simulink library "lib_rfsoc_fec"  (R2020b)
settings: Solver=VariableStepAuto  StartTime=0.0  StopTime=10.0  RelTol=1e-3
undefined symbols (not defined in the file): d, fs, generator_polynomial
libraries: commseqgen3 x84, hdlsllib x83, $bdroot x33, simulink x22, dspsigops x13
(part 2 of 4)

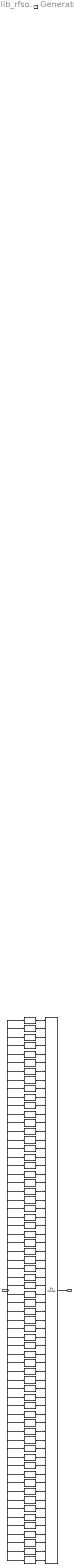
== system lib_rfsoc_fec/Random Number Generator/Random Number Generator ==
  reset : Inport
  enable : EnablePort
  bit0 : commseqgen3/PN Sequence Generator  poly='z^13 + z^12 + z^11 + z^8 + 1'  ini_sta=[ 1 1 1 0 0 1 1 0 0 1 1 0 0]  outBitMaskSource=Dialog parameter  shift=0  outVarSiz=off  maxOutSizeMode=Dialog parameter  maxOutSize=[10 1]  Ts=-1  sampPerFrame=1  reset=on  bitPackedOutputs=off  outDataType=boolean  numPackedBits=8  bitPackDataSigned=off  bitPackedOutDType=double
  bit1 : commseqgen3/PN Sequence Generator  poly='z^13 + z^12 + z^11 + z^8 + 1'  ini_sta=[ 1 0 0 0 0 1 1 0 0 0 1 0 1]  outBitMaskSource=Dialog parameter  shift=0  outVarSiz=off  maxOutSizeMode=Dialog parameter  maxOutSize=[10 1]  Ts=-1  sampPerFrame=1  reset=on  bitPackedOutputs=off  outDataType=boolean  numPackedBits=8  bitPackDataSigned=off  bitPackedOutDType=double
  bit10 : commseqgen3/PN Sequence Generator  poly='z^13 + z^12 + z^11 + z^8 + 1'  ini_sta=[ 1 0 1 0 0 0 1 1 0 1 1 0 0]  outBitMaskSource=Dialog parameter  shift=0  outVarSiz=off  maxOutSizeMode=Dialog parameter  maxOutSize=[10 1]  Ts=-1  sampPerFrame=1  reset=on  bitPackedOutputs=off  outDataType=boolean  numPackedBits=8  bitPackDataSigned=off  bitPackedOutDType=double
  bit11 : commseqgen3/PN Sequence Generator  poly='z^13 + z^12 + z^11 + z^8 + 1'  ini_sta=[ 0 1 0 1 0 1 1 1 1 1 0 1 0]  outBitMaskSource=Dialog parameter  shift=0  outVarSiz=off  maxOutSizeMode=Dialog parameter  maxOutSize=[10 1]  Ts=-1  sampPerFrame=1  reset=on  bitPackedOutputs=off  outDataType=boolean  numPackedBits=8  bitPackDataSigned=off  bitPackedOutDType=double
  bit12 : commseqgen3/PN Sequence Generator  poly='z^13 + z^12 + z^11 + z^8 + 1'  ini_sta=[ 0 0 1 1 0 1 1 1 0 1 1 1 0]  outBitMaskSource=Dialog parameter  shift=0  outVarSiz=off  maxOutSizeMode=Dialog parameter  maxOutSize=[10 1]  Ts=-1  sampPerFrame=1  reset=on  bitPackedOutputs=off  outDataType=boolean  numPackedBits=8  bitPackDataSigned=off  bitPackedOutDType=double
  bit13 : commseqgen3/PN Sequence Generator  poly='z^13 + z^12 + z^11 + z^8 + 1'  ini_sta=[ 1 1 0 0 1 0 0 1 0 1 0 0 0]  outBitMaskSource=Dialog parameter  shift=0  outVarSiz=off  maxOutSizeMode=Dialog parameter  maxOutSize=[10 1]  Ts=-1  sampPerFrame=1  reset=on  bitPackedOutputs=off  outDataType=boolean  numPackedBits=8  bitPackDataSigned=off  bitPackedOutDType=double
  bit14 : commseqgen3/PN Sequence Generator  poly='z^13 + z^12 + z^11 + z^8 + 1'  ini_sta=[ 1 0 1 1 1 0 0 1 0 0 0 1 1]  outBitMaskSource=Dialog parameter  shift=0  outVarSiz=off  maxOutSizeMode=Dialog parameter  maxOutSize=[10 1]  Ts=-1  sampPerFrame=1  reset=on  bitPackedOutputs=off  outDataType=boolean  numPackedBits=8  bitPackDataSigned=off  bitPackedOutDType=double
  bit15 : commseqgen3/PN Sequence Generator  poly='z^13 + z^12 + z^11 + z^8 + 1'  ini_sta=[ 0 1 0 0 0 1 1 1 0 1 1 0 0]  outBitMaskSource=Dialog parameter  shift=0  outVarSiz=off  maxOutSizeMode=Dialog parameter  maxOutSize=[10 1]  Ts=-1  sampPerFrame=1  reset=on  bitPackedOutputs=off  outDataType=boolean  numPackedBits=8  bitPackDataSigned=off  bitPackedOutDType=double
  bit16 : commseqgen3/PN Sequence Generator  poly='z^13 + z^12 + z^11 + z^8 + 1'  ini_sta=[ 1 0 0 1 0 1 0 1 0 0 0 1 1]  outBitMaskSource=Dialog parameter  shift=0  outVarSiz=off  maxOutSizeMode=Dialog parameter  maxOutSize=[10 1]  Ts=-1  sampPerFrame=1  reset=on  bitPackedOutputs=off  outDataType=boolean  numPackedBits=8  bitPackDataSigned=off  bitPackedOutDType=double
  bit17 : commseqgen3/PN Sequence Generator  poly='z^13 + z^12 + z^11 + z^8 + 1'  ini_sta=[ 0 1 1 0 1 0 1 1 1 1 0 0 1]  outBitMaskSource=Dialog parameter  shift=0  outVarSiz=off  maxOutSizeMode=Dialog parameter  maxOutSize=[10 1]  Ts=-1  sampPerFrame=1  reset=on  bitPackedOutputs=off  outDataType=boolean  numPackedBits=8  bitPackDataSigned=off  bitPackedOutDType=double
  bit18 : commseqgen3/PN Sequence Generator  poly='z^13 + z^12 + z^11 + z^8 + 1'  ini_sta=[ 0 0 0 1 0 1 1 1 1 0 0 1 1]  outBitMaskSource=Dialog parameter  shift=0  outVarSiz=off  maxOutSizeMode=Dialog parameter  maxOutSize=[10 1]  Ts=-1  sampPerFrame=1  reset=on  bitPackedOutputs=off  outDataType=boolean  numPackedBits=8  bitPackDataSigned=off  bitPackedOutDType=double
  bit19 : commseqgen3/PN Sequence Generator  poly='z^13 + z^12 + z^11 + z^8 + 1'  ini_sta=[ 0 0 0 0 0 1 1 0 0 0 1 0 1]  outBitMaskSource=Dialog parameter  shift=0  outVarSiz=off  maxOutSizeMode=Dialog parameter  maxOutSize=[10 1]  Ts=-1  sampPerFrame=1  reset=on  bitPackedOutputs=off  outDataType=boolean  numPackedBits=8  bitPackDataSigned=off  bitPackedOutDType=double
  bit2 : commseqgen3/PN Sequence Generator  poly='z^13 + z^12 + z^11 + z^8 + 1'  ini_sta=[ 0 0 0 1 1 1 1 0 1 1 0 0 1]  outBitMaskSource=Dialog parameter  shift=0  outVarSiz=off  maxOutSizeMode=Dialog parameter  maxOutSize=[10 1]  Ts=-1  sampPerFrame=1  reset=on  bitPackedOutputs=off  outDataType=boolean  numPackedBits=8  bitPackDataSigned=off  bitPackedOutDType=double
  bit20 : commseqgen3/PN Sequence Generator  poly='z^13 + z^12 + z^11 + z^8 + 1'  ini_sta=[ 0 1 1 1 1 1 0 1 1 0 1 1 1]  outBitMaskSource=Dialog parameter  shift=0  outVarSiz=off  maxOutSizeMode=Dialog parameter  maxOutSize=[10 1]  Ts=-1  sampPerFrame=1  reset=on  bitPackedOutputs=off  outDataType=boolean  numPackedBits=8  bitPackDataSigned=off  bitPackedOutDType=double
  bit21 : commseqgen3/PN Sequence Generator  poly='z^13 + z^12 + z^11 + z^8 + 1'  ini_sta=[ 0 1 0 0 0 1 1 1 0 1 0 0 0]  outBitMaskSource=Dialog parameter  shift=0  outVarSiz=off  maxOutSizeMode=Dialog parameter  maxOutSize=[10 1]  Ts=-1  sampPerFrame=1  reset=on  bitPackedOutputs=off  outDataType=boolean  numPackedBits=8  bitPackDataSigned=off  bitPackedOutDType=double
  bit22 : commseqgen3/PN Sequence Generator  poly='z^13 + z^12 + z^11 + z^8 + 1'  ini_sta=[ 0 1 0 1 0 1 1 0 1 1 1 1 1]  outBitMaskSource=Dialog parameter  shift=0  outVarSiz=off  maxOutSizeMode=Dialog parameter  maxOutSize=[10 1]  Ts=-1  sampPerFrame=1  reset=on  bitPackedOutputs=off  outDataType=boolean  numPackedBits=8  bitPackDataSigned=off  bitPackedOutDType=double
  bit23 : commseqgen3/PN Sequence Generator  poly='z^13 + z^12 + z^11 + z^8 + 1'  ini_sta=[ 0 1 0 0 1 0 0 1 1 0 0 1 0]  outBitMaskSource=Dialog parameter  shift=0  outVarSiz=off  maxOutSizeMode=Dialog parameter  maxOutSize=[10 1]  Ts=-1  sampPerFrame=1  reset=on  bitPackedOutputs=off  outDataType=boolean  numPackedBits=8  bitPackDataSigned=off  bitPackedOutDType=double
  bit24 : commseqgen3/PN Sequence Generator  poly='z^13 + z^12 + z^11 + z^8 + 1'  ini_sta=[ 0 0 1 0 1 0 1 1 1 1 0 0 0]  outBitMaskSource=Dialog parameter  shift=0  outVarSiz=off  maxOutSizeMode=Dialog parameter  maxOutSize=[10 1]  Ts=-1  sampPerFrame=1  reset=on  bitPackedOutputs=off  outDataType=boolean  numPackedBits=8  bitPackDataSigned=off  bitPackedOutDType=double
  bit25 : commseqgen3/PN Sequence Generator  poly='z^13 + z^12 + z^11 + z^8 + 1'  ini_sta=[ 0 1 1 0 0 1 1 0 0 0 1 1 1]  outBitMaskSource=Dialog parameter  shift=0  outVarSiz=off  maxOutSizeMode=Dialog parameter  maxOutSize=[10 1]  Ts=-1  sampPerFrame=1  reset=on  bitPackedOutputs=off  outDataType=boolean  numPackedBits=8  bitPackDataSigned=off  bitPackedOutDType=double
  bit26 : commseqgen3/PN Sequence Generator  poly='z^13 + z^12 + z^11 + z^8 + 1'  ini_sta=[ 1 0 1 1 0 0 1 0 1 0 0 1 1]  outBitMaskSource=Dialog parameter  shift=0  outVarSiz=off  maxOutSizeMode=Dialog parameter  maxOutSize=[10 1]  Ts=-1  sampPerFrame=1  reset=on  bitPackedOutputs=off  outDataType=boolean  numPackedBits=8  bitPackDataSigned=off  bitPackedOutDType=double
  bit27 : commseqgen3/PN Sequence Generator  poly='z^13 + z^12 + z^11 + z^8 + 1'  ini_sta=[ 0 0 1 1 0 1 0 0 0 0 1 0 1]  outBitMaskSource=Dialog parameter  shift=0  outVarSiz=off  maxOutSizeMode=Dialog parameter  maxOutSize=[10 1]  Ts=-1  sampPerFrame=1  reset=on  bitPackedOutputs=off  outDataType=boolean  numPackedBits=8  bitPackDataSigned=off  bitPackedOutDType=double
  bit28 : commseqgen3/PN Sequence Generator  poly='z^13 + z^12 + z^11 + z^8 + 1'  ini_sta=[ 1 0 1 0 1 0 1 0 1 0 0 1 0]  outBitMaskSource=Dialog parameter  shift=0  outVarSiz=off  maxOutSizeMode=Dialog parameter  maxOutSize=[10 1]  Ts=-1  sampPerFrame=1  reset=on  bitPackedOutputs=off  outDataType=boolean  numPackedBits=8  bitPackDataSigned=off  bitPackedOutDType=double
  bit29 : commseqgen3/PN Sequence Generator  poly='z^13 + z^12 + z^11 + z^8 + 1'  ini_sta=[ 0 1 1 1 0 0 0 1 0 1 1 1 0]  outBitMaskSource=Dialog parameter  shift=0  outVarSiz=off  maxOutSizeMode=Dialog parameter  maxOutSize=[10 1]  Ts=-1  sampPerFrame=1  reset=on  bitPackedOutputs=off  outDataType=boolean  numPackedBits=8  bitPackDataSigned=off  bitPackedOutDType=double
  bit3 : commseqgen3/PN Sequence Generator  poly='z^13 + z^12 + z^11 + z^8 + 1'  ini_sta=[ 0 0 1 0 1 1 0 1 1 0 0 0 1]  outBitMaskSource=Dialog parameter  shift=0  outVarSiz=off  maxOutSizeMode=Dialog parameter  maxOutSize=[10 1]  Ts=-1  sampPerFrame=1  reset=on  bitPackedOutputs=off  outDataType=boolean  numPackedBits=8  bitPackDataSigned=off  bitPackedOutDType=double
  bit30 : commseqgen3/PN Sequence Generator  poly='z^13 + z^12 + z^11 + z^8 + 1'  ini_sta=[ 0 1 1 0 1 1 1 0 1 1 1 1 0]  outBitMaskSource=Dialog parameter  shift=0  outVarSiz=off  maxOutSizeMode=Dialog parameter  maxOutSize=[10 1]  Ts=-1  sampPerFrame=1  reset=on  bitPackedOutputs=off  outDataType=boolean  numPackedBits=8  bitPackDataSigned=off  bitPackedOutDType=double
  bit31 : commseqgen3/PN Sequence Generator  poly='z^13 + z^12 + z^11 + z^8 + 1'  ini_sta=[ 0 0 1 0 1 1 0 0 1 1 1 0 0]  outBitMaskSource=Dialog parameter  shift=0  outVarSiz=off  maxOutSizeMode=Dialog parameter  maxOutSize=[10 1]  Ts=-1  sampPerFrame=1  reset=on  bitPackedOutputs=off  outDataType=boolean  numPackedBits=8  bitPackDataSigned=off  bitPackedOutDType=double
  bit32 : commseqgen3/PN Sequence Generator  poly='z^13 + z^12 + z^11 + z^8 + 1'  ini_sta=[ 0 0 1 1 0 0 0 1 0 1 1 1 1]  outBitMaskSource=Dialog parameter  shift=0  outVarSiz=off  maxOutSizeMode=Dialog parameter  maxOutSize=[10 1]  Ts=-1  sampPerFrame=1  reset=on  bitPackedOutputs=off  outDataType=boolean  numPackedBits=8  bitPackDataSigned=off  bitPackedOutDType=double
  bit33 : commseqgen3/PN Sequence Generator  poly='z^13 + z^12 + z^11 + z^8 + 1'  ini_sta=[ 1 0 0 1 1 1 0 1 1 1 0 1 0]  outBitMaskSource=Dialog parameter  shift=0  outVarSiz=off  maxOutSizeMode=Dialog parameter  maxOutSize=[10 1]  Ts=-1  sampPerFrame=1  reset=on  bitPackedOutputs=off  outDataType=boolean  numPackedBits=8  bitPackDataSigned=off  bitPackedOutDType=double
  bit34 : commseqgen3/PN Sequence Generator  poly='z^13 + z^12 + z^11 + z^8 + 1'  ini_sta=[ 0 1 0 0 0 1 0 0 1 1 1 0 0]  outBitMaskSource=Dialog parameter  shift=0  outVarSiz=off  maxOutSizeMode=Dialog parameter  maxOutSize=[10 1]  Ts=-1  sampPerFrame=1  reset=on  bitPackedOutputs=off  outDataType=boolean  numPackedBits=8  bitPackDataSigned=off  bitPackedOutDType=double
  bit35 : commseqgen3/PN Sequence Generator  poly='z^13 + z^12 + z^11 + z^8 + 1'  ini_sta=[ 1 0 0 0 1 1 1 1 0 1 0 0 1]  outBitMaskSource=Dialog parameter  shift=0  outVarSiz=off  maxOutSizeMode=Dialog parameter  maxOutSize=[10 1]  Ts=-1  sampPerFrame=1  reset=on  bitPackedOutputs=off  outDataType=boolean  numPackedBits=8  bitPackDataSigned=off  bitPackedOutDType=double
  bit36 : commseqgen3/PN Sequence Generator  poly='z^13 + z^12 + z^11 + z^8 + 1'  ini_sta=[ 1 1 1 1 0 0 0 1 1 1 0 1 1]  outBitMaskSource=Dialog parameter  shift=0  outVarSiz=off  maxOutSizeMode=Dialog parameter  maxOutSize=[10 1]  Ts=-1  sampPerFrame=1  reset=on  bitPackedOutputs=off  outDataType=boolean  numPackedBits=8  bitPackDataSigned=off  bitPackedOutDType=double
  bit37 : commseqgen3/PN Sequence Generator  poly='z^13 + z^12 + z^11 + z^8 + 1'  ini_sta=[ 1 0 1 1 0 1 1 0 1 1 1 0 1]  outBitMaskSource=Dialog parameter  shift=0  outVarSiz=off  maxOutSizeMode=Dialog parameter  maxOutSize=[10 1]  Ts=-1  sampPerFrame=1  reset=on  bitPackedOutputs=off  outDataType=boolean  numPackedBits=8  bitPackDataSigned=off  bitPackedOutDType=double
  bit38 : commseqgen3/PN Sequence Generator  poly='z^13 + z^12 + z^11 + z^8 + 1'  ini_sta=[ 1 0 1 0 1 1 0 1 1 1 1 0 0]  outBitMaskSource=Dialog parameter  shift=0  outVarSiz=off  maxOutSizeMode=Dialog parameter  maxOutSize=[10 1]  Ts=-1  sampPerFrame=1  reset=on  bitPackedOutputs=off  outDataType=boolean  numPackedBits=8  bitPackDataSigned=off  bitPackedOutDType=double
  bit39 : commseqgen3/PN Sequence Generator  poly='z^13 + z^12 + z^11 + z^8 + 1'  ini_sta=[ 1 1 1 1 0 1 0 1 1 0 0 1 1]  outBitMaskSource=Dialog parameter  shift=0  outVarSiz=off  maxOutSizeMode=Dialog parameter  maxOutSize=[10 1]  Ts=-1  sampPerFrame=1  reset=on  bitPackedOutputs=off  outDataType=boolean  numPackedBits=8  bitPackDataSigned=off  bitPackedOutDType=double
  bit4 : commseqgen3/PN Sequence Generator  poly='z^13 + z^12 + z^11 + z^8 + 1'  ini_sta=[ 1 0 1 1 0 1 0 0 1 1 0 0 0]  outBitMaskSource=Dialog parameter  shift=0  outVarSiz=off  maxOutSizeMode=Dialog parameter  maxOutSize=[10 1]  Ts=-1  sampPerFrame=1  reset=on  bitPackedOutputs=off  outDataType=boolean  numPackedBits=8  bitPackDataSigned=off  bitPackedOutDType=double
  bit40 : commseqgen3/PN Sequence Generator  poly='z^13 + z^12 + z^11 + z^8 + 1'  ini_sta=[ 1 1 0 0 0 1 1 0 0 1 1 1 1]  outBitMaskSource=Dialog parameter  shift=0  outVarSiz=off  maxOutSizeMode=Dialog parameter  maxOutSize=[10 1]  Ts=-1  sampPerFrame=1  reset=on  bitPackedOutputs=off  outDataType=boolean  numPackedBits=8  bitPackDataSigned=off  bitPackedOutDType=double
  bit41 : commseqgen3/PN Sequence Generator  poly='z^13 + z^12 + z^11 + z^8 + 1'  ini_sta=[ 1 0 0 1 1 0 1 1 1 0 0 1 0]  outBitMaskSource=Dialog parameter  shift=0  outVarSiz=off  maxOutSizeMode=Dialog parameter  maxOutSize=[10 1]  Ts=-1  sampPerFrame=1  reset=on  bitPackedOutputs=off  outDataType=boolean  numPackedBits=8  bitPackDataSigned=off  bitPackedOutDType=double
  bit42 : commseqgen3/PN Sequence Generator  poly='z^13 + z^12 + z^11 + z^8 + 1'  ini_sta=[ 1 1 1 1 0 0 1 0 1 0 1 1 0]  outBitMaskSource=Dialog parameter  shift=0  outVarSiz=off  maxOutSizeMode=Dialog parameter  maxOutSize=[10 1]  Ts=-1  sampPerFrame=1  reset=on  bitPackedOutputs=off  outDataType=boolean  numPackedBits=8  bitPackDataSigned=off  bitPackedOutDType=double
  bit43 : commseqgen3/PN Sequence Generator  poly='z^13 + z^12 + z^11 + z^8 + 1'  ini_sta=[ 0 0 0 0 1 1 1 1 0 1 0 0 1]  outBitMaskSource=Dialog parameter  shift=0  outVarSiz=off  maxOutSizeMode=Dialog parameter  maxOutSize=[10 1]  Ts=-1  sampPerFrame=1  reset=on  bitPackedOutputs=off  outDataType=boolean  numPackedBits=8  bitPackDataSigned=off  bitPackedOutDType=double
  bit44 : commseqgen3/PN Sequence Generator  poly='z^13 + z^12 + z^11 + z^8 + 1'  ini_sta=[ 0 1 0 0 0 1 0 0 1 1 0 1 0]  outBitMaskSource=Dialog parameter  shift=0  outVarSiz=off  maxOutSizeMode=Dialog parameter  maxOutSize=[10 1]  Ts=-1  sampPerFrame=1  reset=on  bitPackedOutputs=off  outDataType=boolean  numPackedBits=8  bitPackDataSigned=off  bitPackedOutDType=double
  bit45 : commseqgen3/PN Sequence Generator  poly='z^13 + z^12 + z^11 + z^8 + 1'  ini_sta=[ 1 1 1 1 1 1 0 0 1 0 0 1 0]  outBitMaskSource=Dialog parameter  shift=0  outVarSiz=off  maxOutSizeMode=Dialog parameter  maxOutSize=[10 1]  Ts=-1  sampPerFrame=1  reset=on  bitPackedOutputs=off  outDataType=boolean  numPackedBits=8  bitPackDataSigned=off  bitPackedOutDType=double
  bit46 : commseqgen3/PN Sequence Generator  poly='z^13 + z^12 + z^11 + z^8 + 1'  ini_sta=[ 1 1 0 0 0 1 0 1 1 0 1 1 0]  outBitMaskSource=Dialog parameter  shift=0  outVarSiz=off  maxOutSizeMode=Dialog parameter  maxOutSize=[10 1]  Ts=-1  sampPerFrame=1  reset=on  bitPackedOutputs=off  outDataType=boolean  numPackedBits=8  bitPackDataSigned=off  bitPackedOutDType=double
  bit47 : commseqgen3/PN Sequence Generator  poly='z^13 + z^12 + z^11 + z^8 + 1'  ini_sta=[ 0 1 1 1 1 0 0 1 1 0 1 1 0]  outBitMaskSource=Dialog parameter  shift=0  outVarSiz=off  maxOutSizeMode=Dialog parameter  maxOutSize=[10 1]  Ts=-1  sampPerFrame=1  reset=on  bitPackedOutputs=off  outDataType=boolean  numPackedBits=8  bitPackDataSigned=off  bitPackedOutDType=double
  bit48 : commseqgen3/PN Sequence Generator  poly='z^13 + z^12 + z^11 + z^8 + 1'  ini_sta=[ 1 0 1 0 1 1 1 0 0 1 0 1 0]  outBitMaskSource=Dialog parameter  shift=0  outVarSiz=off  maxOutSizeMode=Dialog parameter  maxOutSize=[10 1]  Ts=-1  sampPerFrame=1  reset=on  bitPackedOutputs=off  outDataType=boolean  numPackedBits=8  bitPackDataSigned=off  bitPackedOutDType=double
  bit49 : commseqgen3/PN Sequence Generator  poly='z^13 + z^12 + z^11 + z^8 + 1'  ini_sta=[ 0 1 1 0 1 0 1 0 1 1 0 0 0]  outBitMaskSource=Dialog parameter  shift=0  outVarSiz=off  maxOutSizeMode=Dialog parameter  maxOutSize=[10 1]  Ts=-1  sampPerFrame=1  reset=on  bitPackedOutputs=off  outDataType=boolean  numPackedBits=8  bitPackDataSigned=off  bitPackedOutDType=double
  bit5 : commseqgen3/PN Sequence Generator  poly='z^13 + z^12 + z^11 + z^8 + 1'  ini_sta=[ 1 1 0 1 0 1 0 0 1 1 0 1 0]  outBitMaskSource=Dialog parameter  shift=0  outVarSiz=off  maxOutSizeMode=Dialog parameter  maxOutSize=[10 1]  Ts=-1  sampPerFrame=1  reset=on  bitPackedOutputs=off  outDataType=boolean  numPackedBits=8  bitPackDataSigned=off  bitPackedOutDType=double
  bit50 : commseqgen3/PN Sequence Generator  poly='z^13 + z^12 + z^11 + z^8 + 1'  ini_sta=[ 0 1 1 0 0 0 0 1 0 1 0 1 0]  outBitMaskSource=Dialog parameter  shift=0  outVarSiz=off  maxOutSizeMode=Dialog parameter  maxOutSize=[10 1]  Ts=-1  sampPerFrame=1  reset=on  bitPackedOutputs=off  outDataType=boolean  numPackedBits=8  bitPackDataSigned=off  bitPackedOutDType=double
  bit51 : commseqgen3/PN Sequence Generator  poly='z^13 + z^12 + z^11 + z^8 + 1'  ini_sta=[ 0 0 1 1 0 1 1 0 1 0 0 1 1]  outBitMaskSource=Dialog parameter  shift=0  outVarSiz=off  maxOutSizeMode=Dialog parameter  maxOutSize=[10 1]  Ts=-1  sampPerFrame=1  reset=on  bitPackedOutputs=off  outDataType=boolean  numPackedBits=8  bitPackDataSigned=off  bitPackedOutDType=double
  bit52 : commseqgen3/PN Sequence Generator  poly='z^13 + z^12 + z^11 + z^8 + 1'  ini_sta=[ 0 1 1 0 0 0 1 0 0 0 0 0 1]  outBitMaskSource=Dialog parameter  shift=0  outVarSiz=off  maxOutSizeMode=Dialog parameter  maxOutSize=[10 1]  Ts=-1  sampPerFrame=1  reset=on  bitPackedOutputs=off  outDataType=boolean  numPackedBits=8  bitPackDataSigned=off  bitPackedOutDType=double
  bit53 : commseqgen3/PN Sequence Generator  poly='z^13 + z^12 + z^11 + z^8 + 1'  ini_sta=[ 0 0 0 0 0 1 1 1 1 0 1 0 0]  outBitMaskSource=Dialog parameter  shift=0  outVarSiz=off  maxOutSizeMode=Dialog parameter  maxOutSize=[10 1]  Ts=-1  sampPerFrame=1  reset=on  bitPackedOutputs=off  outDataType=boolean  numPackedBits=8  bitPackDataSigned=off  bitPackedOutDType=double
  bit54 : commseqgen3/PN Sequence Generator  poly='z^13 + z^12 + z^11 + z^8 + 1'  ini_sta=[ 0 1 1 1 1 0 0 0 1 1 1 0 1]  outBitMaskSource=Dialog parameter  shift=0  outVarSiz=off  maxOutSizeMode=Dialog parameter  maxOutSize=[10 1]  Ts=-1  sampPerFrame=1  reset=on  bitPackedOutputs=off  outDataType=boolean  numPackedBits=8  bitPackDataSigned=off  bitPackedOutDType=double
  bit55 : commseqgen3/PN Sequence Generator  poly='z^13 + z^12 + z^11 + z^8 + 1'  ini_sta=[ 0 1 0 1 0 1 0 1 0 1 0 1 1]  outBitMaskSource=Dialog parameter  shift=0  outVarSiz=off  maxOutSizeMode=Dialog parameter  maxOutSize=[10 1]  Ts=-1  sampPerFrame=1  reset=on  bitPackedOutputs=off  outDataType=boolean  numPackedBits=8  bitPackDataSigned=off  bitPackedOutDType=double
  bit56 : commseqgen3/PN Sequence Generator  poly='z^13 + z^12 + z^11 + z^8 + 1'  ini_sta=[ 1 1 1 1 1 0 0 1 1 1 0 1 0]  outBitMaskSource=Dialog parameter  shift=0  outVarSiz=off  maxOutSizeMode=Dialog parameter  maxOutSize=[10 1]  Ts=-1  sampPerFrame=1  reset=on  bitPackedOutputs=off  outDataType=boolean  numPackedBits=8  bitPackDataSigned=off  bitPackedOutDType=double
  bit57 : commseqgen3/PN Sequence Generator  poly='z^13 + z^12 + z^11 + z^8 + 1'  ini_sta=[ 1 0 0 0 1 1 1 0 0 0 1 1 0]  outBitMaskSource=Dialog parameter  shift=0  outVarSiz=off  maxOutSizeMode=Dialog parameter  maxOutSize=[10 1]  Ts=-1  sampPerFrame=1  reset=on  bitPackedOutputs=off  outDataType=boolean  numPackedBits=8  bitPackDataSigned=off  bitPackedOutDType=double
  bit58 : commseqgen3/PN Sequence Generator  poly='z^13 + z^12 + z^11 + z^8 + 1'  ini_sta=[ 1 1 0 1 1 0 0 0 1 0 1 0 1]  outBitMaskSource=Dialog parameter  shift=0  outVarSiz=off  maxOutSizeMode=Dialog parameter  maxOutSize=[10 1]  Ts=-1  sampPerFrame=1  reset=on  bitPackedOutputs=off  outDataType=boolean  numPackedBits=8  bitPackDataSigned=off  bitPackedOutDType=double
  bit59 : commseqgen3/PN Sequence Generator  poly='z^13 + z^12 + z^11 + z^8 + 1'  ini_sta=[ 0 1 1 0 1 0 0 0 0 1 1 1 1]  outBitMaskSource=Dialog parameter  shift=0  outVarSiz=off  maxOutSizeMode=Dialog parameter  maxOutSize=[10 1]  Ts=-1  sampPerFrame=1  reset=on  bitPackedOutputs=off  outDataType=boolean  numPackedBits=8  bitPackDataSigned=off  bitPackedOutDType=double
  bit6 : commseqgen3/PN Sequence Generator  poly='z^13 + z^12 + z^11 + z^8 + 1'  ini_sta=[ 0 0 0 0 1 0 0 0 1 1 1 1 0]  outBitMaskSource=Dialog parameter  shift=0  outVarSiz=off  maxOutSizeMode=Dialog parameter  maxOutSize=[10 1]  Ts=-1  sampPerFrame=1  reset=on  bitPackedOutputs=off  outDataType=boolean  numPackedBits=8  bitPackDataSigned=off  bitPackedOutDType=double
  bit60 : commseqgen3/PN Sequence Generator  poly='z^13 + z^12 + z^11 + z^8 + 1'  ini_sta=[ 0 1 1 1 0 1 1 0 0 1 0 0 1]  outBitMaskSource=Dialog parameter  shift=0  outVarSiz=off  maxOutSizeMode=Dialog parameter  maxOutSize=[10 1]  Ts=-1  sampPerFrame=1  reset=on  bitPackedOutputs=off  outDataType=boolean  numPackedBits=8  bitPackDataSigned=off  bitPackedOutDType=double
  bit61 : commseqgen3/PN Sequence Generator  poly='z^13 + z^12 + z^11 + z^8 + 1'  ini_sta=[ 1 1 0 1 0 0 1 1 1 0 0 0 1]  outBitMaskSource=Dialog parameter  shift=0  outVarSiz=off  maxOutSizeMode=Dialog parameter  maxOutSize=[10 1]  Ts=-1  sampPerFrame=1  reset=on  bitPackedOutputs=off  outDataType=boolean  numPackedBits=8  bitPackDataSigned=off  bitPackedOutDType=double
  bit62 : commseqgen3/PN Sequence Generator  poly='z^13 + z^12 + z^11 + z^8 + 1'  ini_sta=[ 1 1 1 1 1 1 0 1 1 0 1 1 1]  outBitMaskSource=Dialog parameter  shift=0  outVarSiz=off  maxOutSizeMode=Dialog parameter  maxOutSize=[10 1]  Ts=-1  sampPerFrame=1  reset=on  bitPackedOutputs=off  outDataType=boolean  numPackedBits=8  bitPackDataSigned=off  bitPackedOutDType=double
  bit63 : commseqgen3/PN Sequence Generator  poly='z^13 + z^12 + z^11 + z^8 + 1'  ini_sta=[ 1 0 0 0 0 1 1 0 0 0 1 0 0]  outBitMaskSource=Dialog parameter  shift=0  outVarSiz=off  maxOutSizeMode=Dialog parameter  maxOutSize=[10 1]  Ts=-1  sampPerFrame=1  reset=on  bitPackedOutputs=off  outDataType=boolean  numPackedBits=8  bitPackDataSigned=off  bitPackedOutDType=double
  bit7 : commseqgen3/PN Sequence Generator  poly='z^13 + z^12 + z^11 + z^8 + 1'  ini_sta=[ 1 1 0 0 0 0 1 0 0 0 0 0 0]  outBitMaskSource=Dialog parameter  shift=0  outVarSiz=off  maxOutSizeMode=Dialog parameter  maxOutSize=[10 1]  Ts=-1  sampPerFrame=1  reset=on  bitPackedOutputs=off  outDataType=boolean  numPackedBits=8  bitPackDataSigned=off  bitPackedOutDType=double
  bit8 : commseqgen3/PN Sequence Generator  poly='z^13 + z^12 + z^11 + z^8 + 1'  ini_sta=[ 1 1 1 1 0 1 0 1 0 0 0 0 0]  outBitMaskSource=Dialog parameter  shift=0  outVarSiz=off  maxOutSizeMode=Dialog parameter  maxOutSize=[10 1]  Ts=-1  sampPerFrame=1  reset=on  bitPackedOutputs=off  outDataType=boolean  numPackedBits=8  bitPackDataSigned=off  bitPackedOutDType=double
  bit9 : commseqgen3/PN Sequence Generator  poly='z^13 + z^12 + z^11 + z^8 + 1'  ini_sta=[ 0 1 0 1 0 1 1 1 1 1 0 0 1]  outBitMaskSource=Dialog parameter  shift=0  outVarSiz=off  maxOutSizeMode=Dialog parameter  maxOutSize=[10 1]  Ts=-1  sampPerFrame=1  reset=on  bitPackedOutputs=off  outDataType=boolean  numPackedBits=8  bitPackDataSigned=off  bitPackedOutDType=double
  concat : hdlsllib/Logic and Bit Operations/Bit Concat  numInputs=64
  data : Outport
  wires:
  concat/1 -> data/1
  bit63/1 -> concat/64
  bit62/1 -> concat/63
  bit61/1 -> concat/62
  bit60/1 -> concat/61
  bit59/1 -> concat/60
  bit58/1 -> concat/59
  bit57/1 -> concat/58
  bit56/1 -> concat/57
  bit55/1 -> concat/56
  bit54/1 -> concat/55
  bit53/1 -> concat/54
  bit52/1 -> concat/53
  bit51/1 -> concat/52
  bit50/1 -> concat/51
  bit49/1 -> concat/50
  bit48/1 -> concat/49
  bit47/1 -> concat/48
  bit46/1 -> concat/47
  bit45/1 -> concat/46
  bit44/1 -> concat/45
  bit43/1 -> concat/44
  bit42/1 -> concat/43
  bit41/1 -> concat/42
  bit40/1 -> concat/41
  bit39/1 -> concat/40
  bit38/1 -> concat/39
  bit37/1 -> concat/38
  bit36/1 -> concat/37
  bit35/1 -> concat/36
  bit34/1 -> concat/35
  bit33/1 -> concat/34
  bit32/1 -> concat/33
  bit31/1 -> concat/32
  bit30/1 -> concat/31
  bit29/1 -> concat/30
  bit28/1 -> concat/29
  bit27/1 -> concat/28
  bit26/1 -> concat/27
  bit25/1 -> concat/26
  bit24/1 -> concat/25
  bit23/1 -> concat/24
  bit22/1 -> concat/23
  bit21/1 -> concat/22
  bit20/1 -> concat/21
  bit19/1 -> concat/20
  bit18/1 -> concat/19
  bit17/1 -> concat/18
  bit16/1 -> concat/17
  bit15/1 -> concat/16
  bit14/1 -> concat/15
  bit13/1 -> concat/14
  bit12/1 -> concat/13
  bit11/1 -> concat/12
  bit10/1 -> concat/11
  bit9/1 -> concat/10
  bit8/1 -> concat/9
  bit7/1 -> concat/8
  bit6/1 -> concat/7
  bit5/1 -> concat/6
  bit4/1 -> concat/5
  bit3/1 -> concat/4
  bit2/1 -> concat/3
  bit1/1 -> concat/2
  bit0/1 -> concat/1
  reset/1 -> bit63/1, bit62/1, bit61/1, bit60/1, bit59/1, bit58/1, bit57/1, bit56/1, bit55/1, bit54/1, bit53/1, bit52/1, bit51/1, bit50/1, bit49/1, bit48/1, bit47/1, bit46/1, bit45/1, bit44/1, bit43/1, bit42/1, bit41/1, bit40/1, bit39/1, bit38/1, bit37/1, bit36/1, bit35/1, bit34/1, bit33/1, bit32/1, bit31/1, bit30/1, bit29/1, bit28/1, bit27/1, bit26/1, bit25/1, bit24/1, bit23/1, bit22/1, bit21/1, bit20/1, bit19/1, bit18/1, bit17/1, bit16/1, bit15/1, bit14/1, bit13/1, bit12/1, bit11/1, bit10/1, bit9/1, bit8/1, bit7/1, bit6/1, bit5/1, bit4/1, bit3/1, bit2/1, bit1/1, bit0/1

== system lib_rfsoc_fec/Random Number Generator/byte_count ==
  reset : Inport
  en : Inport  Port=2
  Cast To Boolean : DataTypeConversion  OutDataTypeStr=boolean
  Delay3 : Delay  DelayLength=1
  Delay5 : Delay  DelayLength=1
  HDL Counter : hdlsllib/Sources/HDL Counter  CountType=Count limited  CountInit=0  CountStep=1  CountMax=1  CountFromType=Initial value  CountFrom=0  CountResetPort=on  CountLoadPort=off  CountEnbPort=on  CountDirPort=off  CountDataType=Unsigned  CountWordLen=1  CountFracLen=0  CountSampTime=1
  HDL Counter1 : hdlsllib/Sources/HDL Counter  CountType=Count limited  CountInit=0  CountStep=1  CountMax=3  CountFromType=Initial value  CountFrom=0  CountResetPort=on  CountLoadPort=off  CountEnbPort=on  CountDirPort=off  CountDataType=Unsigned  CountWordLen=2  CountFracLen=0  CountSampTime=1
  OR : Logic  Operator=OR  IconShape=distinctive  AllPortsSameDT=off  OutDataTypeStr=boolean
  falling_edge : Subsystem
  count : Outport
  valid : Outport  Port=2
  wires:
  Cast To Boolean/1 -> HDL Counter1/2, valid/1
  falling_edge/1(pulse) -> OR/2
  Delay3/1 -> OR/1
  HDL Counter1/1 -> count/1
  reset/1 -> Delay3/1
  Delay5/1 -> HDL Counter/2, falling_edge/1(in)
  HDL Counter/1 -> Cast To Boolean/1
  OR/1 -> HDL Counter/1, HDL Counter1/1
  en/1 -> Delay5/1

== system lib_rfsoc_fec/Random Number Generator/concat ==
  en : Inport
  d_in : Inport  Port=2
  diff : Inport  Port=3
  Bit Concat : hdlsllib/Logic and Bit Operations/Bit Concat  numInputs=2
  Bitwise Operator : simulink/Logic and Bit Operations/Bitwise Operator  logicop=AND  UseBitMask=off  NumInputPorts=2  BitMask=bin2dec('11011001')  BitMaskRealWorld=Stored Integer
  Constant : Constant  Value=0  OutDataTypeStr=fixdt(0,128,0)  SampleTime=-1
  Delay : Delay  DelayLength=1
  Delay1 : Delay  DelayLength=1
  Delay4 : Delay  DelayLength=1
  Multiport Switch : MultiPortSwitch  DataPortOrder=Zero-based contiguous  Inputs=2  zeroidx=on
  mask_generator : Subsystem
  d_out : Outport
  wires:
  Delay/1 -> Multiport Switch/1
  Constant/1 -> Multiport Switch/2
  Bitwise Operator/1 -> Multiport Switch/3
  en/1 -> mask_generator/2(sel), Delay/1
  Multiport Switch/1 -> d_out/1
  mask_generator/1(mask) -> Bitwise Operator/2
  Delay1/1 -> Bitwise Operator/1
  diff/1 -> mask_generator/1(diff)
  Bit Concat/1 -> Delay1/1
  d_in/1 -> Delay4/1, Bit Concat/1
  Delay4/1 -> Bit Concat/2

== system lib_rfsoc_fec/Random Number Generator/hold for multiple of 4 ==
  In1 : Inport
  Compare To Constant : simulink/Logic and Bit Operations/Compare To Constant  relop===  const=7  OutDataTypeStr=boolean
  HDL Counter : hdlsllib/Sources/HDL Counter  CountType=Count limited  CountInit=0  CountStep=1  CountMax=7  CountFromType=Initial value  CountFrom=0  CountResetPort=off  CountLoadPort=off  CountEnbPort=on  CountDirPort=off  CountDataType=Unsigned  CountWordLen=3  CountFracLen=0  CountSampTime=1
  OR : Logic  Operator=OR  IconShape=distinctive  AllPortsSameDT=off  OutDataTypeStr=boolean
  Sample and Hold1 : dspsigops/Sample and Hold  trig=Rising edge  initCond=0  latchinput=off
  " " : Outport
  wires:
  Compare To Constant/1 -> OR/1
  HDL Counter/1 -> Compare To Constant/1
  OR/1 -> Sample and Hold1/Trigger
  Sample and Hold1/1 -> " "/1, HDL Counter/1
  In1/1 -> Sample and Hold1/1, OR/2

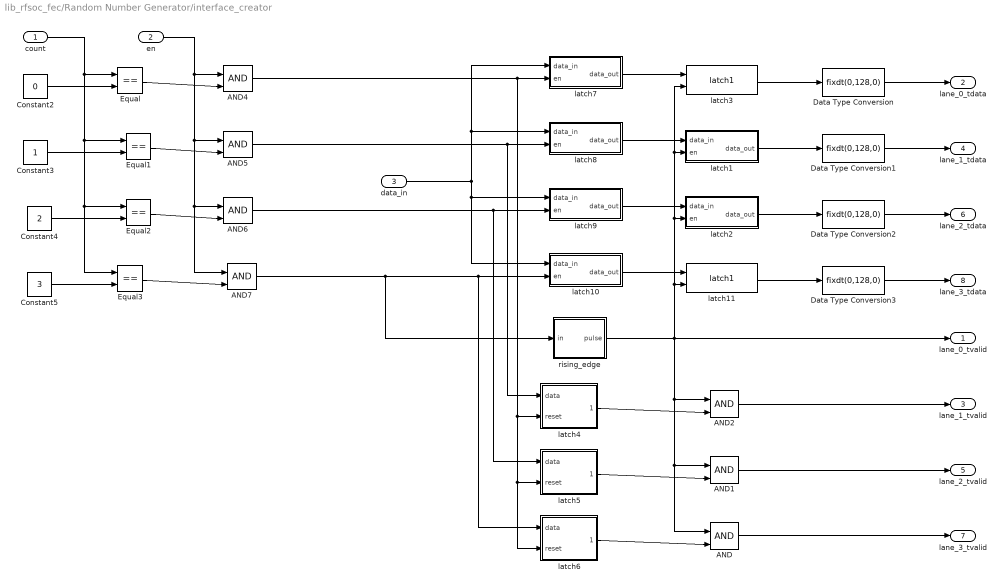
== system lib_rfsoc_fec/Random Number Generator/interface_creator ==
  count : Inport
  en : Inport  Port=2
  data_in : Inport  Port=3
  AND{,1..2,4..7} (7 alike) : Logic  IconShape=distinctive  AllPortsSameDT=off  OutDataTypeStr=boolean
  Constant2 : Constant  Value=0  OutDataTypeStr=fixdt(0,2,0)  SampleTime=-1
  Constant3 : Constant  OutDataTypeStr=fixdt(0,2,0)  SampleTime=-1
  Constant4 : Constant  Value=2  OutDataTypeStr=fixdt(0,2,0)  SampleTime=-1
  Constant5 : Constant  Value=3  OutDataTypeStr=fixdt(0,2,0)  SampleTime=-1
  Data Type Conversion{,1..3} (4 alike) : DataTypeConversion  OutDataTypeStr=fixdt(0,128,0)
  Equal{,1..3} (4 alike) : RelationalOperator  Operator===  OutDataTypeStr=boolean  RndMeth=Simplest
  latch1 : Subsystem
  latch10 : Subsystem
  latch11 : $bdroot/Random Number Generator/interface_creator/latch1  SystemSampleTime=-1  VariantActivationTime=update diagram  Latency=0  AutoFrameSizeCalculation=off
  latch2 : Subsystem
  latch3 : $bdroot/Random Number Generator/interface_creator/latch1  SystemSampleTime=-1  VariantActivationTime=update diagram  Latency=0  AutoFrameSizeCalculation=off
  latch4 : Subsystem
  latch5 : Subsystem
  latch6 : Subsystem
  latch7 : Subsystem
  latch8 : Subsystem
  latch9 : Subsystem
  rising_edge : Subsystem
  lane_0_tvalid : Outport
  lane_0_tdata : Outport  Port=2
  lane_1_tvalid : Outport  Port=3
  lane_1_tdata : Outport  Port=4
  lane_2_tvalid : Outport  Port=5
  lane_2_tdata : Outport  Port=6
  lane_3_tvalid : Outport  Port=7
  lane_3_tdata : Outport  Port=8
  wires:
  AND/1 -> lane_3_tvalid/1
  latch2/1(data_out) -> Data Type Conversion2/1
  latch6/1(data_out) -> AND/2
  AND7/1 -> latch6/1(data), latch10/2(en), rising_edge/1(in)
  latch4/1(data_out) -> AND2/2
  Constant3/1 -> Equal1/2
  latch10/1(data_out) -> latch11/1
  latch1/1(data_out) -> Data Type Conversion1/1
  Equal/1 -> AND4/2
  Equal1/1 -> AND5/2
  latch5/1(data_out) -> AND1/2
  AND1/1 -> lane_2_tvalid/1
  Equal2/1 -> AND6/2
  rising_edge/1(pulse) -> AND2/1, AND1/1, AND/1, latch11/2, latch2/2(en), latch3/2, latch1/2(en), lane_0_tvalid/1
  Constant2/1 -> Equal/2
  latch11/1 -> Data Type Conversion3/1
  latch7/1(data_out) -> latch3/1
  AND4/1 -> latch7/2(en), latch4/2(reset), latch5/2(reset), latch6/2(reset)
  latch9/1(data_out) -> latch2/1(data_in)
  en/1 -> AND4/1, AND7/1, AND6/1, AND5/1
  Constant5/1 -> Equal3/2
  Constant4/1 -> Equal2/2
  AND5/1 -> latch4/1(data), latch8/2(en)
  AND6/1 -> latch5/1(data), latch9/2(en)
  AND2/1 -> lane_1_tvalid/1
  latch8/1(data_out) -> latch1/1(data_in)
  data_in/1 -> latch8/1(data_in), latch7/1(data_in), latch9/1(data_in), latch10/1(data_in)
  latch3/1 -> Data Type Conversion/1
  Equal3/1 -> AND7/2
  count/1 -> Equal/1, Equal1/1, Equal2/1, Equal3/1
  Data Type Conversion/1 -> lane_0_tdata/1
  Data Type Conversion1/1 -> lane_1_tdata/1
  Data Type Conversion2/1 -> lane_2_tdata/1
  Data Type Conversion3/1 -> lane_3_tdata/1

== system lib_rfsoc_fec/Random Number Generator/rising_edge ==
  in : Inport
  Data Type Conversion1 : DataTypeConversion  OutDataTypeStr=boolean  SaturateOnIntegerOverflow=on  RndMeth=Zero
  Delay15 : Delay  DelayLength=1  InitialCondition=1  InputProcessing=Columns as channels (frame based)
  Logical Operator2 : Logic  Operator=NOT  Inputs=1
  Logical Operator3 : Logic
  pulse : Outport
  wires:
  Logical Operator2/1 -> Logical Operator3/2
  in/1 -> Data Type Conversion1/1
  Data Type Conversion1/1 -> Logical Operator3/1, Delay15/1
  Logical Operator3/1 -> pulse/1
  Delay15/1 -> Logical Operator2/1

== system lib_rfsoc_fec/Random Number Generator/tvalid hold ==
  trigger : Inport
  comparator : Inport  Port=2
  Cast To Boolean : DataTypeConversion  OutDataTypeStr=boolean
  Delay2 : Delay  DelayLength=1
  Equal : RelationalOperator  OutDataTypeStr=boolean  RndMeth=Simplest
  HDL Counter : hdlsllib/Sources/HDL Counter  CountType=Free running  CountInit=0  CountStep=128  CountMax=25  CountFromType=Initial value  CountFrom=0  CountResetPort=on  CountLoadPort=off  CountEnbPort=on  CountDirPort=off  CountDataType=Unsigned  CountWordLen=32  CountFracLen=0  CountSampTime=1
  HDL Counter1 : hdlsllib/Sources/HDL Counter  CountType=Count limited  CountInit=0  CountStep=1  CountMax=1  CountFromType=Initial value  CountFrom=0  CountResetPort=on  CountLoadPort=off  CountEnbPort=on  CountDirPort=off  CountDataType=Unsigned  CountWordLen=1  CountFracLen=0  CountSampTime=1
  Multiport Switch : MultiPortSwitch  DataPortOrder=Zero-based contiguous  Inputs=2  zeroidx=on
  OR : Logic  Operator=OR  IconShape=distinctive  AllPortsSameDT=off  OutDataTypeStr=boolean
  Subtract : Sum  Inputs=+-
  enable : Outport
  diff : Outport  Port=2
  wires:
  Cast To Boolean/1 -> HDL Counter/2
  HDL Counter1/1 -> Cast To Boolean/1
  Subtract/1 -> diff/1
  HDL Counter/1 -> Equal/1, Subtract/1
  Equal/1 -> HDL Counter/1, HDL Counter1/1, OR/1
  trigger/1 -> Multiport Switch/3, OR/2
  comparator/1 -> Equal/2, Subtract/2
  Multiport Switch/1 -> Delay2/1, HDL Counter1/2, enable/1
  Delay2/1 -> Multiport Switch/2
  OR/1 -> Multiport Switch/1

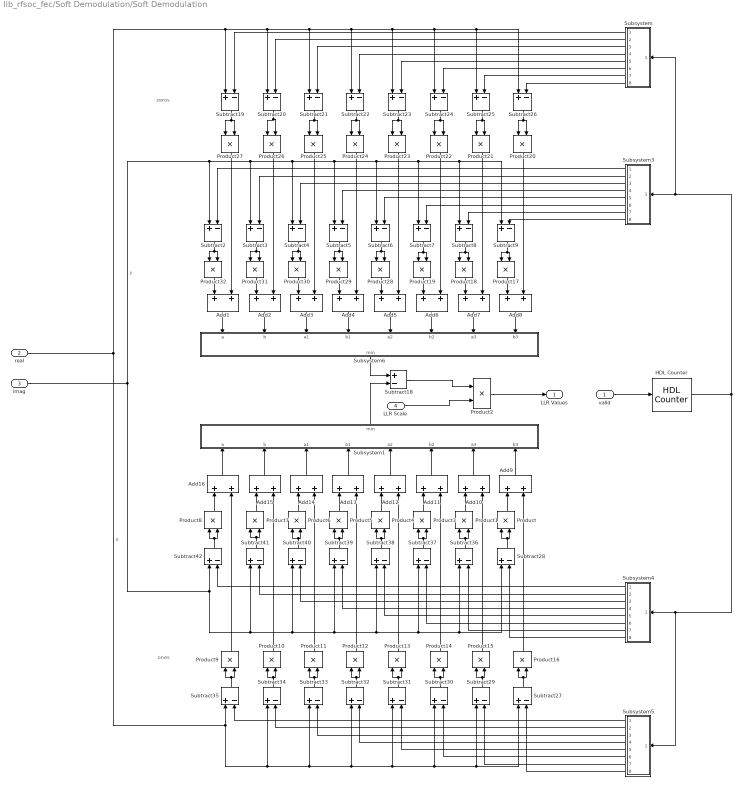
== system lib_rfsoc_fec/Soft Demodulation/Soft Demodulation ==
  note: ones
  note: zeros
  valid : Inport
  real : Inport  Port=2
  imag : Inport  Port=3
  LLR Scale : Inport  Port=4
  Add{1..16} (16 alike) : Sum  OutDataTypeStr=fixdt(1,35,22)  SaturateOnIntegerOverflow=on
  HDL Counter : hdlsllib/Sources/HDL Counter  CountType=Count limited  CountInit=0  CountStep=1  CountMax=3  CountFromType=Initial value  CountFrom=0  CountResetPort=off  CountLoadPort=off  CountEnbPort=on  CountDirPort=off  CountDataType=Unsigned  CountWordLen=2  CountFracLen=0  CountSampTime=1/(fs*2)
  Product{,1,3..16} (16 alike) : Product  SaturateOnIntegerOverflow=on
  Product{17..32} (16 alike) : Product
  Product2 : Product  OutDataTypeStr=fixdt(1,24,12)  RndMeth=Round  SaturateOnIntegerOverflow=on
  Subsystem : Subsystem
  Subsystem1 : Subsystem
  Subsystem3 : Subsystem
  Subsystem4 : Subsystem
  Subsystem5 : Subsystem
  Subsystem6 : Subsystem
  Subtract18 : Sum  Inputs=+-  OutDataTypeStr=fixdt(1,35,22)  SaturateOnIntegerOverflow=on
  Subtract{2..9,19..42} (32 alike) : Sum  Inputs=+-  OutDataTypeStr=fixdt(1,17,11)  SaturateOnIntegerOverflow=on
  LLR Values : Outport
  wires:
  HDL Counter/1 -> Subsystem3/1(enb), Subsystem/1(enb), Subsystem4/1(enb), Subsystem5/1(enb)
  valid/1 -> HDL Counter/1
  Subsystem/8(Out8) -> Subtract26/2
  Subsystem/7(Out7) -> Subtract25/2
  Subsystem/6(Out6) -> Subtract24/2
  Subsystem/5(Out5) -> Subtract23/2
  Subsystem/4(Out4) -> Subtract22/2
  Subsystem/3(Out3) -> Subtract21/2
  Subsystem/2(Out2) -> Subtract20/2
  Subsystem/1(Out1) -> Subtract19/2
  Subtract7/1 -> Product19/2, Product19/1
  Subtract22/1 -> Product24/2, Product24/1
  Subtract20/1 -> Product26/1, Product26/2
  Subtract8/1 -> Product18/2, Product18/1
  Subtract9/1 -> Product17/1, Product17/2
  Subtract27/1 -> Product16/2, Product16/1
  Subtract29/1 -> Product15/2, Product15/1
  Subtract30/1 -> Product14/2, Product14/1
  Subtract31/1 -> Product13/2, Product13/1
  Subtract32/1 -> Product12/2, Product12/1
  Subtract33/1 -> Product11/2, Product11/1
  Subtract37/1 -> Product3/2, Product3/1
  Product2/1 -> LLR Values/1
  Subsystem5/5(Out5) -> Subtract31/2
  Subtract28/1 -> Product/1, Product/2
  Add5/1 -> Subsystem6/5(a2)
  Subsystem3/8(Out8) -> Subtract9/2
  Add4/1 -> Subsystem6/4(b1)
  Product11/1 -> Add14/2
  Product29/1 -> Add4/1
  Subsystem4/8(Out8) -> Subtract28/2
  Subsystem4/2(Out2) -> Subtract41/2
  Subsystem5/8(Out8) -> Subtract27/2
  Subsystem5/7(Out7) -> Subtract29/2
  Subtract40/1 -> Product6/1, Product6/2
  Subtract34/1 -> Product10/1, Product10/2
  Product32/1 -> Add1/1
  Subsystem5/1(Out1) -> Subtract35/2
  Subtract39/1 -> Product5/1, Product5/2
  Subsystem3/7(Out7) -> Subtract8/2
  Product16/1 -> Add9/2
  Subsystem4/1(Out1) -> Subtract42/2
  Subsystem5/6(Out6) -> Subtract30/2
  Product24/1 -> Add4/2
  Subtract3/1 -> Product31/2, Product31/1
  Product13/1 -> Add12/2
  Subsystem5/3(Out3) -> Subtract33/2
  Subsystem5/2(Out2) -> Subtract34/2
  Subsystem4/3(Out3) -> Subtract40/2
  Product17/1 -> Add8/1
  Subsystem4/4(Out4) -> Subtract39/2
  Product9/1 -> Add16/2
  Add15/1 -> Subsystem1/2(b)
  Subsystem4/7(Out7) -> Subtract36/2
  Subtract26/1 -> Product20/2, Product20/1
  Subsystem3/3(Out3) -> Subtract4/2
  Product28/1 -> Add5/1
  Product12/1 -> Add13/2
  Product8/1 -> Add16/1
  Product7/1 -> Add15/1
  Subsystem4/5(Out5) -> Subtract38/2
  Subsystem3/4(Out4) -> Subtract5/2
  Product21/1 -> Add7/2
  Subtract25/1 -> Product21/2, Product21/1
  Add6/1 -> Subsystem6/6(b2)
  Add13/1 -> Subsystem1/4(b1)
  Add2/1 -> Subsystem6/2(b)
  Product15/1 -> Add10/2
  Product14/1 -> Add11/2
  Add8/1 -> Subsystem6/8(b3)
  Product27/1 -> Add1/2
  Subsystem3/1(Out1) -> Subtract2/2
  Subtract42/1 -> Product8/1, Product8/2
  Subtract36/1 -> Product1/1, Product1/2
  Subtract23/1 -> Product23/1, Product23/2
  Add10/1 -> Subsystem1/7(a3)
  imag/1 -> Subtract42/1, Subtract39/1, Subtract28/1, Subtract36/1, Subtract37/1, Subtract38/1, Subtract40/1, Subtract41/1, Subtract9/1, Subtract8/1, Subtract7/1, Subtract6/1, Subtract5/1, Subtract4/1, Subtract3/1, Subtract2/1  "y"
  Add16/1 -> Subsystem1/1(a)
  Subtract2/1 -> Product32/2, Product32/1
  Subtract6/1 -> Product28/2, Product28/1
  Subtract5/1 -> Product29/1, Product29/2
  Product18/1 -> Add7/1
  Add9/1 -> Subsystem1/8(b3)
  Product30/1 -> Add3/1
  Subsystem3/5(Out5) -> Subtract6/2
  Product31/1 -> Add2/1
  Subtract19/1 -> Product27/2, Product27/1
  Product26/1 -> Add2/2
  Add11/1 -> Subsystem1/6(b2)
  Subsystem3/2(Out2) -> Subtract3/2
  Product22/1 -> Add6/2
  Subsystem1/1(min) -> Subtract18/2
  Product5/1 -> Add13/1
  Subtract18/1 -> Product2/1
  Subsystem4/6(Out6) -> Subtract37/2
  Subtract4/1 -> Product30/2, Product30/1
  Subtract24/1 -> Product22/2, Product22/1
  Add14/1 -> Subsystem1/3(a1)
  LLR Scale/1 -> Product2/2
  Product4/1 -> Add12/1
  Subtract21/1 -> Product25/2, Product25/1
  Product23/1 -> Add5/2
  Add7/1 -> Subsystem6/7(a3)
  Product3/1 -> Add11/1
  Product19/1 -> Add6/1
  Product25/1 -> Add3/2
  real/1 -> Subtract27/1, Subtract29/1, Subtract30/1, Subtract31/1, Subtract32/1, Subtract33/1, Subtract34/1, Subtract35/1, Subtract20/1, Subtract26/1, Subtract25/1, Subtract24/1, Subtract23/1, Subtract22/1, Subtract21/1, Subtract19/1  "X"
  Subtract35/1 -> Product9/1, Product9/2
  Subtract41/1 -> Product7/1, Product7/2
  Subsystem3/6(Out6) -> Subtract7/2
  Subsystem6/1(min) -> Subtract18/1
  Add3/1 -> Subsystem6/3(a1)
  Product20/1 -> Add8/2
  Add1/1 -> Subsystem6/1(a)
  Product/1 -> Add9/1
  Subtract38/1 -> Product4/2, Product4/1
  Product1/1 -> Add10/1
  Add12/1 -> Subsystem1/5(a2)
  Product10/1 -> Add15/2
  Product6/1 -> Add14/1
  Subsystem5/4(Out4) -> Subtract32/2

== system lib_rfsoc_fec/Soft Demodulation/sign_extend ==
  u : Inport
  Bit Concat : hdlsllib/Logic and Bit Operations/Bit Concat  numInputs=3
  Bit Slice : hdlsllib/Logic and Bit Operations/Bit Slice  lidx=5  ridx=5
      settings: SourceProductBaseCode=SL
  y : Outport
  wires:
  Bit Concat/1 -> y/1
  u/1 -> Bit Concat/3, Bit Slice/1
  Bit Slice/1 -> Bit Concat/2, Bit Concat/1
